simulink model "forMaple"  (R2014a)
settings: Solver=ode45  StartTime=0.0  StopTime=10.0  RelTol=1e-3
libraries: simulink x2
settings Model: Creator=yoshi12  LastModifiedBy=yoshi12

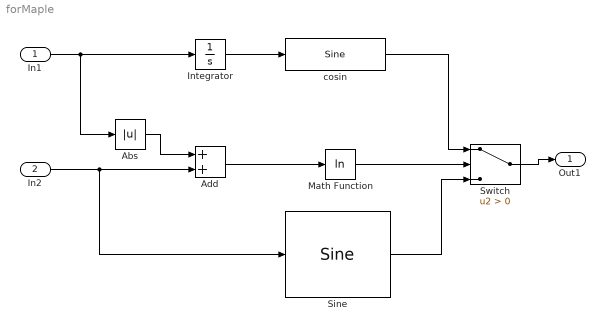
== system forMaple ==
  In1 : Inport
  In2 : Inport  Port=2
  Abs : Abs
  Add : Sum
  Integrator : Integrator
  Math Function : Math  Operator=log  SaturateOnIntegerOverflow=on
  Sine : simulink/Lookup Tables/Sine  Formula=sin(2*pi*u)  NumDataPoints=(2^5)+1  OutputWordLength=16  InternalRulePriority=Speed
  Switch : Switch  Criteria=u2 > Threshold
  cosin : simulink/Lookup Tables/Sine  Formula=cos(2*pi*u)  NumDataPoints=(2^5)+1  OutputWordLength=16  InternalRulePriority=Speed
  Out1 : Outport
  wires:
  In1/1 -> Abs/1, Integrator/1
  Abs/1 -> Add/1
  In2/1 -> Sine/1, Add/2
  Add/1 -> Math Function/1
  Math Function/1 -> Switch/2
  Integrator/1 -> cosin/1
  cosin/1 -> Switch/1
  Sine/1 -> Switch/3
  Switch/1 -> Out1/1
